simulink model "prueba_UDP"  (R2018a)
settings: Solver=VariableStepAuto  StartTime=0.0  StopTime=inf  RelTol=1e-3
undefined symbols (not defined in the file or in its folder): f
libraries: instrumentlib x4
settings Model: Creator=MarioAndres  LastModifiedBy=MarioAndres

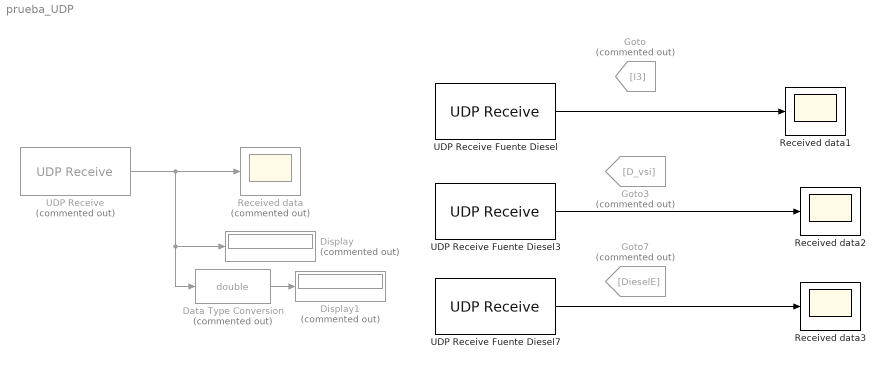
== system prueba_UDP ==
  Data Type Conversion : DataTypeConversion  Commented=on  OutDataTypeStr=double
  Display : Display  Commented=on
  Display1 : Display  Commented=on
  Goto : Goto  Commented=on  GotoTag=I3
  Goto3 : Goto  Commented=on  GotoTag=D_vsi
  Goto7 : Goto  Commented=on  GotoTag=DieselE
  Received data : Scope  Commented=on
      settings: Priority=4
  Received data1 : Scope
      settings: Priority=4
  Received data2 : Scope
      settings: Priority=4
  Received data3 : Scope
      settings: Priority=4
  UDP Receive : instrumentlib/UDP Receive  Priority=3  Commented=on  Host=172.16.49.83  Port=8887  LocalPort=8886  EnablePortSharing=off  GetLatestData=off  DataSize=1  DataType=ASCII  ASCIIFormatting=%f,  Terminator=LF  ByteOrder=BigEndian  EnableBlockingMode=on  Timeout=5  SampleTime=0.1  LocalAddress=0.0.0.0
      settings: SourceProductName=Instrument Control Toolbox
  UDP Receive Fuente Diesel : instrumentlib/UDP Receive  Host=172.16.49.88  Port=8887  LocalPort=8890  EnablePortSharing=off  GetLatestData=off  DataSize=1  DataType=ASCII  ASCIIFormatting=%f,  Terminator=LF  ByteOrder=BigEndian  EnableBlockingMode=on  Timeout=100  SampleTime=-1  LocalAddress=0.0.0.0
      settings: SourceProductName=Instrument Control Toolbox
  UDP Receive Fuente Diesel3 : instrumentlib/UDP Receive  Host=172.16.49.88  Port=8887  LocalPort=8893  EnablePortSharing=off  GetLatestData=off  DataSize=1  DataType=ASCII  ASCIIFormatting=%f,  Terminator=LF  ByteOrder=BigEndian  EnableBlockingMode=on  Timeout=100  SampleTime=-1  LocalAddress=0.0.0.0
      settings: SourceProductName=Instrument Control Toolbox
  UDP Receive Fuente Diesel7 : instrumentlib/UDP Receive  Host=172.16.49.88  Port=8887  LocalPort=8897  EnablePortSharing=off  GetLatestData=off  DataSize=1  DataType=ASCII  ASCIIFormatting=%f,  Terminator=LF  ByteOrder=BigEndian  EnableBlockingMode=on  Timeout=100  SampleTime=-1  LocalAddress=0.0.0.0
      settings: SourceProductName=Instrument Control Toolbox
  wires:
  UDP Receive/1 -> Data Type Conversion/1, Display/1, Received data/1
  Data Type Conversion/1 -> Display1/1
  UDP Receive Fuente Diesel/1 -> Received data1/1
  UDP Receive Fuente Diesel3/1 -> Received data2/1
  UDP Receive Fuente Diesel7/1 -> Received data3/1
